simulink model "g21_final_view_record_pci6221_c_int"  (R2023b)
settings: Solver=ode3  StartTime=0.0  StopTime=20  RelTol=1e-3  EnableMultiTasking=on
values from neighbouring files (symbols this model uses):
  A = sys.A    [g21_script.m]
  B = sys.B    [g21_script.m]
  C = sys.C    [g21_script.m]
  K_cal = [Kp Ke 0 0]    [g21_script.m]
  Nbar = Nu + K * Nx    [g21_script.m]
undefined symbols (not defined in the file or in its folder): DiscIntNeverNeededParam, K, M, National_Instruments, PCI
libraries: sldrtlib x2
settings Model: SimulationMode=external  ExtModeTrigDuration=100000  Creator=Alunos  LastModifiedBy=bernardolopes
settings SolverCC: AlgebraicLoopSolver=TrustRegion
settings DataIOCC: LimitDataPoints=on  SaveFormat=Array  ReturnWorkspaceOutputs=off
settings DebuggingCC: UnconnectedInputMsg=warning  UnconnectedOutputMsg=warning  UnconnectedLineMsg=warning  SFUnexpectedBacktrackingDiag=warning  SFNoUnconditionalDefaultTransitionDiag=warning  SFExecutionAtInitializationDiag=none  ArithmeticOperatorsInVariantConditions=warning
settings HardwareCC: ProdBitPerLong=64  ProdHWDeviceType=Intel->x86-64 (Linux 64)  TargetIntDivRoundTo=Zero  TargetEndianess=LittleEndian  TargetHWDeviceType=Intel->x86/Pentium
settings ModelReferenceCC: PropagateSignalLabelsOutOfModel=off
settings SFSimCC: SimUseLocalCustomCode=off  CustomCodeUndefinedFunction=UseInterfaceOnly
settings RTWCC: Description=Simulink Desktop Real-Time  SystemTargetFile=sldrt.tlc  TemplateMakefile=sldrt.tmf  RTWUseLocalCustomCode=off  RTWCompilerOptimization=on
settings CodeAppCC: MaxIdLength=95  StateflowObjectComments=on
settings SimulinkDesktopRealTimeCC: TargetLibSuffix=_sldrt.a  TargetPreCompLibLocation=C:\Program Files\MATLAB\R2023b\toolbox\sldrt\lib\win64  TargetLangStandard=C89/C90 (ANSI)  SupportVariableSizeSignals=off
settings ConfigComp: CovMetricSettings=dw  CovSaveCumulativeToWorkspaceVar=on  CovSaveSingleToWorkspaceVar=on  CovExternalEMLEnable=off

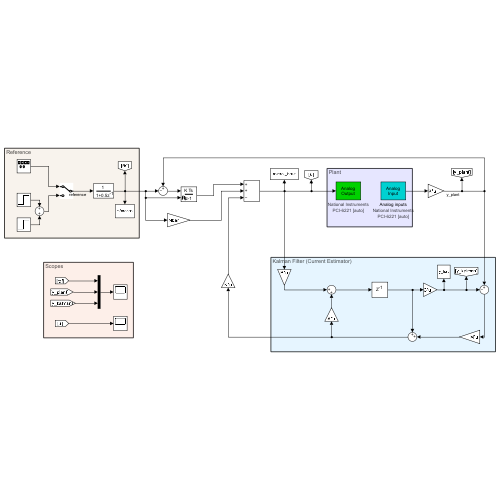
[thumbnail: Simulink's stored preview of the top-level diagram]
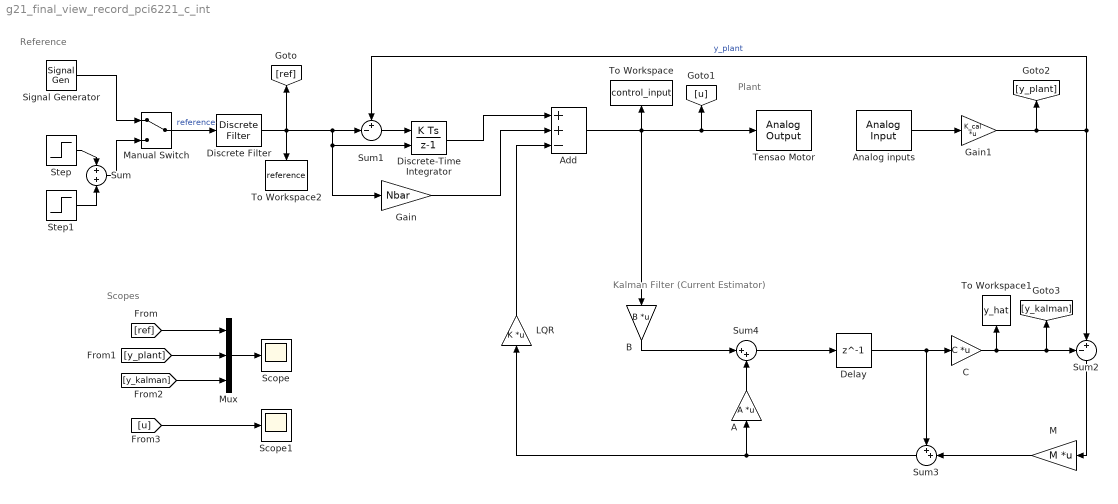
== system g21_final_view_record_pci6221_c_int ==
  note: Scopes
  note: Reference
  note: Plant
  note: Kalman Filter (Current Estimator)
  A : Gain  Gain=A  Multiplication=Matrix(K*u)
  Add : Sum  Inputs=++-
  Analog inputs : sldrtlib/Analog Input  SampleTime=2e-2  MaxMissedTicks=10  ShowMissedTicks=off  YieldWhenWaiting=off  DrvName=National_Instruments/PCI-6221  DrvAddress=4294967295  DrvOptions=[0 0 0 0 0]  Channels=1:4  RangeMode=1  VoltRange=1  DataType=1
      settings: AttributesFormatString=National Instruments\nPCI-6221 [auto]
  B : Gain  Gain=B  Multiplication=Matrix(K*u)
  C : Gain  Gain=C  Multiplication=Matrix(K*u)
  Delay : Delay  DelayLength=1  InitialCondition=0
  Discrete Filter : DiscreteFilter
  Discrete-Time Integrator : DiscreteIntegrator  gainval=0.02  ExternalReset=either  SampleTime=0.02  ICPrevOutput=DiscIntNeverNeededParam  ICPrevScaledInput=DiscIntNeverNeededParam
  Gain : Gain  Gain=Nbar
  Gain1 : Gain  Gain=K_cal  Multiplication=Matrix(K*u)
  LQR : Gain  Gain=K  Multiplication=Matrix(K*u)
  M : Gain  Gain=M  Multiplication=Matrix(K*u)
  Manual Switch : ManualSwitch
  Mux : Mux  Inputs=3
  Scope : Scope
  Scope1 : Scope
  Signal Generator : SignalGenerator  WaveForm=square  Amplitude=30  Frequency=0.2
  Step : Step  Time=2  After=50  SampleTime=0
  Step1 : Step  Time=4  After=0  SampleTime=0
  Sum : Sum  Inputs=+|+
  Sum1 : Sum  Inputs=+-|
  Sum2 : Sum  Inputs=-+|
  Sum3 : Sum  Inputs=++|
  Sum4 : Sum  Inputs=|++
  Tensao Motor : sldrtlib/Analog Output  SampleTime=2e-2  MaxMissedTicks=10  ShowMissedTicks=off  YieldWhenWaiting=off  DrvName=National_Instruments/PCI-6221  DrvAddress=4294967295  DrvOptions=[0 0 0 0 0]  Channels=1  RangeMode=1  VoltRange=1  InitialValue=0  FinalValue=0
      settings: AttributesFormatString=National Instruments\nPCI-6221 [auto]
  To Workspace : ToWorkspace  VariableName=control_input  SampleTime=-1
      settings: Save2DSignal=2-D array (concatenate along first dimension)
  To Workspace1 : ToWorkspace  VariableName=y_hat  SampleTime=-1
      settings: Save2DSignal=2-D array (concatenate along first dimension)
  To Workspace2 : ToWorkspace  VariableName=reference  SampleTime=-1
      settings: Save2DSignal=2-D array (concatenate along first dimension)
  wires:
  Add/1 -> [u], Tensao Motor/1, To Workspace/1, B/1
  Gain1/1 -> Sum2/2, Sum1/1, [y_plant]  "y_plant"
  C/1 -> [y_kalman], Sum2/1, To Workspace1/1
  Sum2/1 -> M/1
  B/1 -> Sum4/1
  Sum3/1 -> A/1, LQR/1
  A/1 -> Sum4/2
  Sum4/1 -> Delay/1
  Delay/1 -> C/1, Sum3/1
  M/1 -> Sum3/2
  Analog inputs/1 -> Gain1/1
  Manual Switch/1 -> Discrete Filter/1  "reference"
  Sum/1 -> Manual Switch/2
  Step1/1 -> Sum/2
  Step/1 -> Sum/1
  Signal Generator/1 -> Manual Switch/1
  Sum1/1 -> Discrete-Time Integrator/1
  Discrete-Time Integrator/1 -> Add/1
  Gain/1 -> Add/2
  LQR/1 -> Add/3
  [y_kalman] -> Mux/3
  Mux/1 -> Scope/1
  [ref] -> Mux/1
  [y_plant] -> Mux/2
  [u] -> Scope1/1
  Discrete Filter/1 -> To Workspace2/1, Gain/1, Discrete-Time Integrator/2, Sum1/2, [ref]
